simulink model "ee"  (R2021b)
settings: Solver=FixedStepAuto  StartTime=0.0  StopTime=10.0  RelTol=1e-3
settings Model: Creator=marco  LastModifiedBy=angelo
settings ConfigComp: DVMode=PropertyProving  DVMaxProcessTime=14400  DVTestSuiteOptimization=Auto  DVDetectOutOfBounds=on  DVMaxViolationSteps=5  DVModelReferenceHarness=on

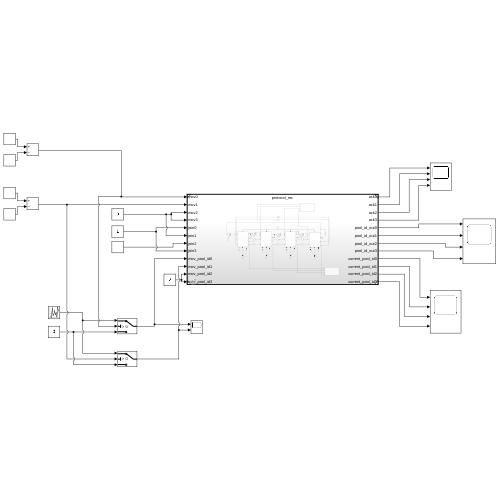
[thumbnail: Simulink's stored preview of the top-level diagram]
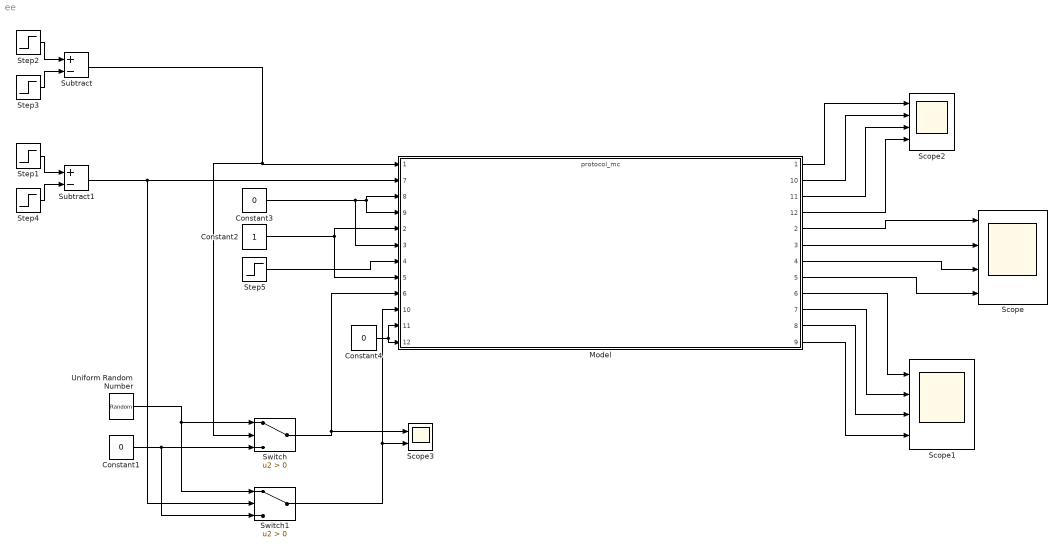
== system ee ==
  Constant1 : Constant  Value=0
  Constant2 : Constant
  Constant3 : Constant  Value=0
  Constant4 : Constant  Value=0
  Model : ModelReference  ModelNameDialog=protocol_mc.slx  SimulationMode=Normal  ModelReferenceVersion=1.165
      settings: PortSchema="{\"entries\":[{\"content\":{\"sides\":[{\"content\":{\"connectorIds\":[\"In1\",\"In7\",\"In8\",\"In9\",\"In2\",\"In3\",\"In4\",\"In5\",\"In6\",\"In10\",\"In11\",\"In12\"]},\"type\":\"ConnectorPlacement.EquallySpacedRectSide\",\"uuid\":\"a8b2226d-44c9-4ce8-8c19-0bc57c3e63cc\"},{\"content\":{\"connectorIds\":[\"Out1\",\"Out10\",\"Out11\",\"Out12\",\"Out2\",\"Out3\",\"Out4\",\"Out5\",\"Out6\",\"Out7\",\"Out8\",\"Out9\"],\"side\":\"RIGHT\"},\"type\":\"ConnectorPlacement.EquallySpacedRectSide\",\"uuid\":\"6850dd4f-634c-44f8-a94c-2056f142a249\"},{\"content\":{\"connectorIds\":[],\"side\":\"TOP\"},\"type\":\"ConnectorPlacement.EquallySpacedRectSide\",\"uuid\":\"db7c17e9-d8fd-4084-957a-a148b3613c07\"}]},\"type\":\"ConnectorPlacement.EquallySpacedConnector\",\"uuid\":\"73dc548a-99fe-4585-b75f-bbc334f72eaf\"}],\"packageUris\":[\"http://schema.mathworks.com/mf0/Connector/R2020b\"],\"version\":\"1.0\"}"
  Scope : Scope  NumInputPorts=4
  Scope1 : Scope  NumInputPorts=4
  Scope2 : Scope  NumInputPorts=4
  Scope3 : Scope  NumInputPorts=2
  Step1 : Step  Time=2.4  SampleTime=.2
  Step2 : Step  SampleTime=.2
  Step3 : Step  Time=1.2  SampleTime=.2
  Step4 : Step  Time=2.6  SampleTime=.2
  Step5 : Step  Time=2.2  SampleTime=.2
  Subtract : Sum  Inputs=+-
  Subtract1 : Sum  Inputs=+-
  Switch : Switch  Criteria=u2 > Threshold
  Switch1 : Switch  Criteria=u2 > Threshold
  Uniform Random Number : UniformRandomNumber  Minimum=1  Maximum=1024  SampleTime=0.2
  wires:
  Step3/1 -> Subtract/2
  Step2/1 -> Subtract/1
  Subtract/1 -> Switch/2, Model/1
  Model/2 -> Scope/1
  Model/3 -> Scope/2
  Model/4 -> Scope/3
  Model/5 -> Scope/4
  Constant1/1 -> Switch1/3, Switch/3
  Switch/1 -> Scope3/1, Model/6
  Constant2/1 -> Model/5, Model/2
  Model/6 -> Scope1/1
  Model/7 -> Scope1/2
  Model/8 -> Scope1/3
  Model/9 -> Scope1/4
  Step1/1 -> Subtract1/1
  Step4/1 -> Subtract1/2
  Model/1 -> Scope2/1
  Subtract1/1 -> Switch1/2, Model/7
  Step5/1 -> Model/4
  Uniform Random Number/1 -> Switch1/1, Switch/1
  Model/10 -> Scope2/2
  Model/11 -> Scope2/3
  Model/12 -> Scope2/4
  Constant3/1 -> Model/3, Model/9, Model/8
  Switch1/1 -> Scope3/2, Model/10
  Constant4/1 -> Model/12, Model/11
